simulink model "mrac"  (Simulink 4.00)
settings: Solver=ode45  StartTime=0.0  StopTime=20.0  MinStep=0.00001  RelTol=1e-5
undefined symbols (not defined in the file): am, ap, bm, bp, gamma
settings Model: LastModifiedBy=gordon

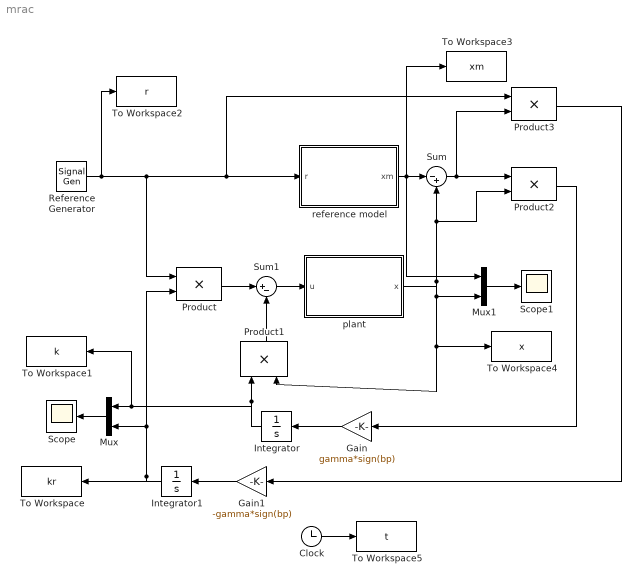
== system mrac ==
  Clock : Clock
      settings: DisplayTime=off  Decimation=10
  Gain : Gain  Orientation=left  Gain=gamma*sign(bp)  Multiplication=Element-wise(K.*u)  SaturateOnIntegerOverflow=on
  Gain1 : Gain  Orientation=left  Gain=-gamma*sign(bp)  Multiplication=Element-wise(K.*u)  SaturateOnIntegerOverflow=on
  Integrator : Integrator  Orientation=left  ExternalReset=none  InitialConditionSource=internal  InitialCondition=1  LimitOutput=off  UpperSaturationLimit=inf  LowerSaturationLimit=-inf  ShowSaturationPort=off  ShowStatePort=off  AbsoluteTolerance=auto
  Integrator1 : Integrator  Orientation=left  ExternalReset=none  InitialConditionSource=internal  InitialCondition=2  LimitOutput=off  UpperSaturationLimit=inf  LowerSaturationLimit=-inf  ShowSaturationPort=off  ShowStatePort=off  AbsoluteTolerance=auto
  Mux : Mux  Orientation=left  Inputs=2
  Mux1 : Mux  Inputs=2
  Product : Product  Inputs=2  Multiplication=Element-wise(.*)  SaturateOnIntegerOverflow=on
  Product1 : Product  Orientation=up  Inputs=2  Multiplication=Element-wise(.*)  SaturateOnIntegerOverflow=on
  Product2 : Product  Inputs=2  Multiplication=Element-wise(.*)  SaturateOnIntegerOverflow=on
  Product3 : Product  Inputs=2  Multiplication=Element-wise(.*)  SaturateOnIntegerOverflow=on
  Reference Generator : SignalGenerator  WaveForm=square  Amplitude=1  Frequency=0.1  Units=Hertz
  Scope : Scope
      settings: TimeRange=auto  YMin=-5  YMax=5  SaveToWorkspace=off  SaveName=ScopeData  MaxDataPoints=5000
  Scope1 : Scope
      settings: TimeRange=auto  YMin=-5  YMax=5  SaveToWorkspace=off  MaxDataPoints=5000
  Sum : Sum  Inputs=|-+  SaturateOnIntegerOverflow=on
  Sum1 : Sum  Inputs=|+-  SaturateOnIntegerOverflow=on
  To Workspace : ToWorkspace  VariableName=kr  SampleTime=-1  SaveFormat=Array
  To Workspace1 : ToWorkspace  VariableName=k  SampleTime=-1  SaveFormat=Array
  To Workspace2 : ToWorkspace  VariableName=r  SampleTime=-1  SaveFormat=Array
  To Workspace3 : ToWorkspace  VariableName=xm  SampleTime=-1  SaveFormat=Array
  To Workspace4 : ToWorkspace  VariableName=x  SampleTime=-1  SaveFormat=Array
  To Workspace5 : ToWorkspace  VariableName=t  SampleTime=-1  SaveFormat=Array
  plant : Subsystem
      settings: RTWFcnNameOpts=Auto  RTWFileNameOpts=Auto
  reference model : Subsystem
      settings: RTWFcnNameOpts=Auto  RTWFileNameOpts=Auto
  wires:
  reference model/1(xm) -> Sum/1, Mux1/1, To Workspace3/1
  plant/1(x) -> Sum/2, Product2/2, Mux1/2, Product1/2, To Workspace4/1
  Product1/1 -> Sum1/2
  Reference Generator/1 -> Product/1, reference model/1(r), Product3/1, To Workspace2/1
  Product/1 -> Sum1/1
  Sum1/1 -> plant/1(u)
  Sum/1 -> Product2/1, Product3/2
  Integrator/1 -> Product1/1, Mux/1, To Workspace1/1
  Integrator1/1 -> Product/2, Mux/2, To Workspace/1
  Gain1/1 -> Integrator1/1
  Gain/1 -> Integrator/1
  Product2/1 -> Gain/1
  Product3/1 -> Gain1/1
  Mux/1 -> Scope/1
  Mux1/1 -> Scope1/1
  Clock/1 -> To Workspace5/1

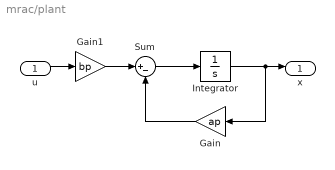
== system mrac/plant ==
  u : Inport  Port=1  LatchInput=off
  Gain : Gain  Orientation=left  Gain=ap  Multiplication=Element-wise(K.*u)  SaturateOnIntegerOverflow=on
  Gain1 : Gain  Gain=bp  Multiplication=Element-wise(K.*u)  SaturateOnIntegerOverflow=on
  Integrator : Integrator  ExternalReset=none  InitialConditionSource=internal  InitialCondition=0  LimitOutput=off  UpperSaturationLimit=inf  LowerSaturationLimit=-inf  ShowSaturationPort=off  ShowStatePort=off  AbsoluteTolerance=auto
  Sum : Sum  Inputs=|+-  SaturateOnIntegerOverflow=on
  x : Outport  Port=1
  wires:
  Gain1/1 -> Sum/1
  Sum/1 -> Integrator/1
  Gain/1 -> Sum/2
  Integrator/1 -> Gain/1, x/1
  u/1 -> Gain1/1

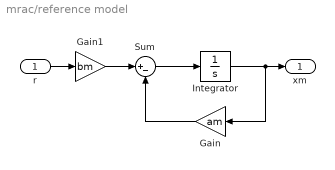
== system mrac/reference model ==
  r : Inport  Port=1  LatchInput=off
  Gain : Gain  Orientation=left  Gain=am  Multiplication=Element-wise(K.*u)  SaturateOnIntegerOverflow=on
  Gain1 : Gain  Gain=bm  Multiplication=Element-wise(K.*u)  SaturateOnIntegerOverflow=on
  Integrator : Integrator  ExternalReset=none  InitialConditionSource=internal  InitialCondition=0  LimitOutput=off  UpperSaturationLimit=inf  LowerSaturationLimit=-inf  ShowSaturationPort=off  ShowStatePort=off  AbsoluteTolerance=auto
  Sum : Sum  Inputs=|+-  SaturateOnIntegerOverflow=on
  xm : Outport  Port=1
  wires:
  r/1 -> Gain1/1
  Integrator/1 -> xm/1, Gain/1
  Gain/1 -> Sum/2
  Sum/1 -> Integrator/1
  Gain1/1 -> Sum/1
